simulink model "sine"  (R2013a)
settings: Solver=ode45  StartTime=0.0  StopTime=10.0  RelTol=1e-3
settings Model: Creator=Sunil  LastModifiedBy=Sunil

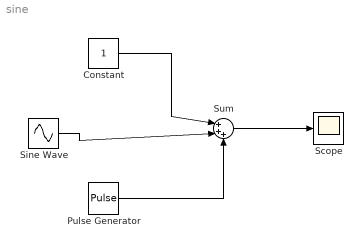
== system sine ==
  Constant : Constant
  Pulse Generator : DiscretePulseGenerator  PulseType=Time based  Period=10  PulseWidth=5
  Scope : Scope
  Sine Wave : Sin  SampleTime=0
  Sum : Sum  Inputs=|+++
  wires:
  Sine Wave/1 -> Sum/2
  Constant/1 -> Sum/1
  Pulse Generator/1 -> Sum/3
  Sum/1 -> Scope/1
